simulink model "pwminverter_c"  (R2019b)
settings: Solver=ode23tb  StartTime=0.0  StopTime=0.2  RelTol=1e-3  EnableMultiTasking=on
libraries: powerlib x50, powerlib_meascontrol x1
settings Model: Creator=g0305973  LastModifiedBy=User
settings DataIOCC: LimitDataPoints=on  SaveFormat=Array  SignalLoggingSaveFormat=ModelDataLogs  ReturnWorkspaceOutputs=off
settings OptimizationCC: ExpressionDepthLimit=2147483647  InitFltsAndDblsToZero=on  LifeSpan=inf
settings DebuggingCC: SaveWithParameterizedLinksMsg=none  UnderspecifiedInitializationDetection=Classic  MergeDetectMultiDrivingBlocksExec=none  SignalResolutionControl=TryResolveAllWithWarning  SolverPrmCheckMsg=warning  FcnCallInpInsideContextMsg=warning  StateNameClashWarn=warning  SFUnexpectedBacktrackingDiag=warning  SFNoUnconditionalDefaultTransitionDiag=warning  SFExecutionAtInitializationDiag=none  ArithmeticOperatorsInVariantConditions=warning
settings HardwareCC: ProdBitPerPointer=32  ProdBitPerSizeT=32  ProdBitPerPtrDiffT=32  ProdLargestAtomicFloat=None  ProdIntDivRoundTo=Undefined  ProdEndianess=Unspecified  ProdWordSize=32  ProdHWDeviceType=32-bit Generic
settings ModelReferenceCC: PropagateSignalLabelsOutOfModel=off
settings SFSimCC: SimUseLocalCustomCode=off  CustomCodeUndefinedFunction=UseInterfaceOnly
settings RTWCC: RTWUseLocalCustomCode=off
settings CodeAppCC: StateflowObjectComments=on
settings GRTTargetCC: TargetFcnLib=ansi_tfl_tmw.mat  TargetLangStandard=C89/C90 (ANSI)  CombineOutputUpdateFcns=off  GRTInterface=on
settings ConfigComp: CovMetricSettings=dw  CovSaveCumulativeToWorkspaceVar=on  CovSaveSingleToWorkspaceVar=on  CovExternalEMLEnable=off
settings SimscapeCC: SimscapeNormalizeSystem=off

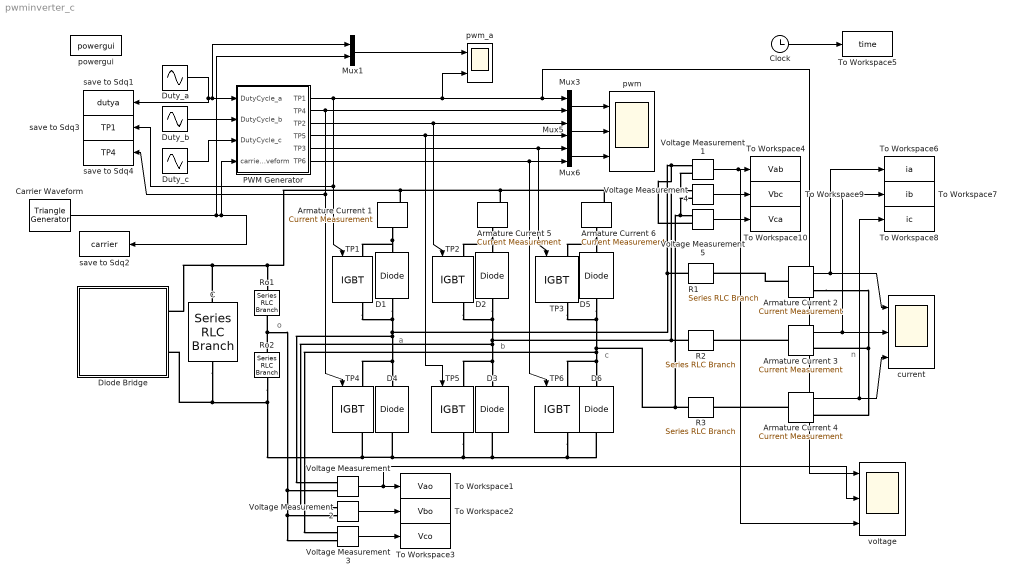
== system pwminverter_c ==
  note: o
  note: n
  note: a
  note: b
  note: c
  Armature Current {1..6} (6 alike) : powerlib/Measurements/Current Measurement  Tag=PoWeRsYsTeMmEaSuReMeNt  PhasorSimulation=off  OutputType=Magnitude  PSBequivalent=0
  C : powerlib/Elements/Series RLC Branch  LConnTagsString=__new0  RConnTagsString=__new0  BranchType=C  Resistance=1.0  Inductance=0.005  SetiL0=off  InitialCurrent=0  Capacitance=100000e-6  Setx0=on  InitialVoltage=390  Measurements=None
  Carrier Waveform : powerlib_meascontrol/Pulse & Signal Generators/Triangle Generator  Freq=2000  Phase=90  Ts=0
  Clock : Clock
  D{1..6} (6 alike) : powerlib/Power Electronics/Diode  Ron=1e-3  Lon=0  Vf=0  IC=0  UseSnubber=off  Rs=1e5  Cs=inf  Measurements=off
  Diode Bridge : Subsystem
  Duty_a : Sin  Amplitude=0.5  Frequency=200*pi  SampleTime=0
  Duty_b : Sin  Amplitude=0.5  Frequency=200*pi  Phase=-2*pi/3  SampleTime=0
  Duty_c : Sin  Amplitude=0.5  Frequency=200*pi  Phase=2*pi/3  SampleTime=0
  Mux{1,3,5..6} (4 alike) : Mux  Inputs=2
  PWM Generator : Subsystem
      mask Display: plot([1,2,2,3,3,4,4,5,5,6],[0,0,5,5,0,0,5,5,0,0])
  R1 : powerlib/Elements/Series RLC Branch  LConnTagsString=__new0  RConnTagsString=__new0  BranchType=RL  Resistance=660  Inductance=1.6  SetiL0=off  InitialCurrent=0  Capacitance=10000e-6  Setx0=off  InitialVoltage=0  Measurements=None
  R2 : powerlib/Elements/Series RLC Branch  LConnTagsString=__new0  RConnTagsString=__new0  BranchType=RL  Resistance=660  Inductance=1.6  SetiL0=off  InitialCurrent=0  Capacitance=10000e-6  Setx0=off  InitialVoltage=0  Measurements=None
  R3 : powerlib/Elements/Series RLC Branch  LConnTagsString=__new0  RConnTagsString=__new0  BranchType=RL  Resistance=660  Inductance=1.6  SetiL0=off  InitialCurrent=0  Capacitance=10000e-6  Setx0=off  InitialVoltage=0  Measurements=None
  Ro1 : powerlib/Elements/Series RLC Branch  LConnTagsString=__new0  RConnTagsString=__new0  BranchType=R  Resistance=4800  Inductance=0.005  SetiL0=off  InitialCurrent=0  Capacitance=10000e-6  Setx0=off  InitialVoltage=0  Measurements=None
  Ro2 : powerlib/Elements/Series RLC Branch  LConnTagsString=__new0  RConnTagsString=__new0  BranchType=R  Resistance=4800  Inductance=0.005  SetiL0=off  InitialCurrent=0  Capacitance=10000e-6  Setx0=off  InitialVoltage=0  Measurements=None
  TP{1..6} (6 alike) : powerlib/Power Electronics/IGBT  Ron=0.001  Lon=0  Vf=0  Tf=1e-6  Tt=2e-6  IC=0  Rs=1e5  Cs=inf  Measurements=on
  To Workspace1 : ToWorkspace  VariableName=Vao  SampleTime=1e-5
  To Workspace10 : ToWorkspace  VariableName=Vca  SampleTime=1e-5
  To Workspace2 : ToWorkspace  VariableName=Vbo  SampleTime=1e-5
  To Workspace3 : ToWorkspace  VariableName=Vco  SampleTime=1e-5
  To Workspace4 : ToWorkspace  VariableName=Vab  SampleTime=1e-5
  To Workspace5 : ToWorkspace  VariableName=time  SampleTime=1e-5
  To Workspace6 : ToWorkspace  VariableName=ia  SampleTime=1e-5
  To Workspace7 : ToWorkspace  VariableName=ib  SampleTime=1e-5
  To Workspace8 : ToWorkspace  VariableName=ic  SampleTime=1e-5
  To Workspace9 : ToWorkspace  VariableName=Vbc  SampleTime=1e-5
  Voltage Measurement{,1..5} (6 alike) : powerlib/Measurements/Voltage Measurement  PhasorSimulation=off  OutputType=Complex  PSBequivalent=0
  current : Scope  NumInputPorts=3
  powergui : powerlib/powergui  SimulationMode=Continuous  SampleTime=50e-6  frequency=60  Iterations=50  frequencyindice=50  Pbase=100e6  ErrMax=1e-4  UnitsV=kV  UnitsW=MW  buscounter=0  FunctionMessages=off  echomessages=off  EnableUseOfTLC=off  CurrentSourceSwitches=on  DisableSnubberDevices=off  DisableRonSwitches=off  DisableVfSwitches=off  DisplayEquations=off  AutomaticDiscreteSolvers=off  SolverType=Tustin  Interpol=off  ExternalGateDelay=off  methode=off  Ts=0  x0status=blocks  SPID=off  SwTol=0  HookPort=off  NonlinearTolerance=1e-4  nMaxIteration=100  ContinueOnMaxIteration=off  RestoreLinks=warning  ResistiveCurrentMeasurement=off  Frange=[0:2:500]  Ylog=off  Xlog=on  ShowGrid=off  save=off  variable=ZData  structure=PhaseCurrent  ZoomFFT=on  StartTime=0.0  cycles=10  DisplayStyle=1  fundamental=100  FreqAxis=off  MaxFrequency=3000  frequencyindicesteady=1  RmsSteady=1  display=off
  pwm : Scope  NumInputPorts=3
  pwm_a : Scope  NumInputPorts=2
  save to Sdq1 : ToWorkspace  VariableName=dutya  SampleTime=1e-5
  save to Sdq2 : ToWorkspace  VariableName=carrier  SampleTime=1e-5
  save to Sdq3 : ToWorkspace  VariableName=TP1  SampleTime=1e-5
  save to Sdq4 : ToWorkspace  VariableName=TP4  SampleTime=1e-5
  voltage : Scope  NumInputPorts=3
  wires:
  Clock/1 -> To Workspace5/1
  PWM Generator/1(TP1) -> Mux3/1, voltage/1, pwm_a/2, TP1/1, save to Sdq3/1
  PWM Generator/2(TP4) -> Mux3/2, TP4/1, save to Sdq4/1
  PWM Generator/3(TP2) -> Mux5/1, TP2/1
  PWM Generator/4(TP5) -> Mux5/2, TP5/1
  PWM Generator/5(TP3) -> Mux6/1, TP3/1
  PWM Generator/6(TP6) -> Mux6/2, TP6/1
  Duty_b/1 -> PWM Generator/2(DutyCycle_b)
  Duty_a/1 -> PWM Generator/1(DutyCycle_a), Mux1/1, save to Sdq1/1
  Duty_c/1 -> PWM Generator/3(DutyCycle_c)
  Mux3/1 -> pwm/1
  Mux5/1 -> pwm/2
  Mux6/1 -> pwm/3
  Voltage Measurement1/1 -> voltage/3, To Workspace4/1
  Voltage Measurement/1 -> voltage/2, To Workspace1/1
  Carrier Waveform/1 -> save to Sdq2/1, PWM Generator/4(carrier waveform), Mux1/2
  Mux1/1 -> pwm_a/1
  Voltage Measurement2/1 -> To Workspace2/1
  Voltage Measurement3/1 -> To Workspace3/1
  Armature Current 3/1 -> current/2, To Workspace7/1
  Armature Current 4/1 -> current/3, To Workspace8/1
  Voltage Measurement4/1 -> To Workspace9/1
  Voltage Measurement5/1 -> To Workspace10/1
  Armature Current 2/1 -> current/1, To Workspace6/1
  connections:
  Armature Current 2/LConn1 -- R1/LConn1
  Armature Current 3/LConn1 -- R2/LConn1
  Armature Current 4/LConn1 -- R3/LConn1
  Armature Current 2/RConn1 -- Armature Current 3/RConn1 -- Armature Current 4/RConn1
  Ro2/LConn1 -- Ro1/RConn1 -- Voltage Measurement/LConn2 -- Voltage Measurement2/LConn2 -- Voltage Measurement3/LConn2
  R3/RConn1 -- TP3/RConn1 -- D5/LConn1 -- TP6/LConn1 -- D6/RConn1 -- Voltage Measurement3/LConn1 -- Voltage Measurement4/LConn2 -- Voltage Measurement5/LConn1
  R2/RConn1 -- TP2/RConn1 -- D2/LConn1 -- D3/RConn1 -- TP5/LConn1 -- Voltage Measurement2/LConn1 -- Voltage Measurement1/LConn2 -- Voltage Measurement4/LConn1
  R1/RConn1 -- TP4/LConn1 -- D4/RConn1 -- Voltage Measurement/LConn1 -- TP1/RConn1 -- D1/LConn1 -- Voltage Measurement5/LConn2 -- Voltage Measurement1/LConn1
  D5/RConn1 -- Armature Current 6/LConn1 -- TP3/LConn1
  D2/RConn1 -- Armature Current 5/LConn1 -- TP2/LConn1
  Armature Current 6/RConn1 -- C/LConn1 -- Diode Bridge/LConn1 -- Ro1/LConn1 -- Armature Current 1/RConn1 -- Armature Current 5/RConn1
  TP1/LConn1 -- Armature Current 1/LConn1 -- D1/RConn1
  C/RConn1 -- Diode Bridge/LConn2 -- D4/LConn1 -- TP5/RConn1 -- TP6/RConn1 -- D6/LConn1 -- D3/LConn1 -- TP4/RConn1 -- Ro2/RConn1

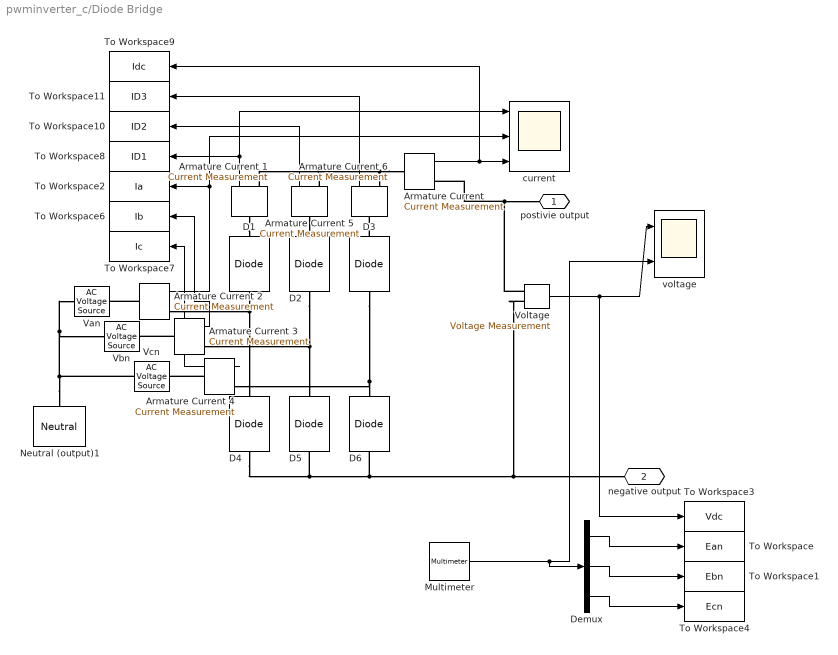
== system pwminverter_c/Diode Bridge ==
  Armature Current {,1..6} (7 alike) : powerlib/Measurements/Current Measurement  Tag=PoWeRsYsTeMmEaSuReMeNt  PhasorSimulation=off  OutputType=Magnitude  PSBequivalent=0
  D{1..6} (6 alike) : powerlib/Power Electronics/Diode  Ron=1e-3  Lon=0  Vf=0  IC=0  UseSnubber=off  Rs=1e5  Cs=inf  Measurements=off
  Demux : Demux  Outputs=3
      settings: DisplayOption=none
  Multimeter : powerlib/Measurements/Multimeter  PhasorSimulation=off  OutputType=Complex  sel=[1 2 3]  L=3  Gain=[1 1 1]  yselected={'Usrc: Diode Bridge/Van','Usrc: Diode Bridge/Vbn','Usrc: Diode Bridge/Vcn'};  PSBOutputType=1  PSBequivalent=0  AxesSetting=[0,0.1,-100,100]  Display=0  SavedBlockNames=-11
  Neutral (output)1 : powerlib/Elements/Neutral  LConnTagsString=a  NodeNumber=99
      settings: SourceProductBaseCode=PS
  To Workspace : ToWorkspace  VariableName=Ean  SampleTime=1e-4
  To Workspace1 : ToWorkspace  VariableName=Ebn  SampleTime=1e-4
  To Workspace10 : ToWorkspace  VariableName=ID2  SampleTime=1e-4
  To Workspace11 : ToWorkspace  VariableName=ID3  SampleTime=1e-4
  To Workspace2 : ToWorkspace  VariableName=Ia  SampleTime=1e-4
  To Workspace3 : ToWorkspace  VariableName=Vdc  SampleTime=1e-4
  To Workspace4 : ToWorkspace  VariableName=Ecn  SampleTime=1e-4
  To Workspace6 : ToWorkspace  VariableName=Ib  SampleTime=1e-4
  To Workspace7 : ToWorkspace  VariableName=Ic  SampleTime=1e-4
  To Workspace8 : ToWorkspace  VariableName=ID1  SampleTime=1e-4
  To Workspace9 : ToWorkspace  VariableName=Idc  SampleTime=1e-4
  Van : powerlib/Electrical Sources/AC Voltage Source  Description=source block  Amplitude=240*1.414  Phase=0  Frequency=50  SampleTime=0  Measurements=Voltage  BusType=swing  Pref=10e3  Qref=0  Qmin=-inf  Qmax=+inf
      settings: AttributesFormatString=\n
  Vbn : powerlib/Electrical Sources/AC Voltage Source  Description=source block  Amplitude=240*1.414  Phase=-120  Frequency=50  SampleTime=0  Measurements=Voltage  BusType=swing  Pref=10e3  Qref=0  Qmin=-inf  Qmax=+inf
      settings: AttributesFormatString=\n
  Vcn : powerlib/Electrical Sources/AC Voltage Source  Description=source block  Amplitude=240*1.414  Phase=120  Frequency=50  SampleTime=0  Measurements=Voltage  BusType=swing  Pref=10e3  Qref=0  Qmin=-inf  Qmax=+inf
      settings: AttributesFormatString=\n
  "Voltage " : powerlib/Measurements/Voltage Measurement  PhasorSimulation=off  OutputType=Complex  PSBequivalent=0
  current : Scope  NumInputPorts=3
  voltage : Scope  NumInputPorts=2
  postivie output : PMIOPort  Side=Left
  negative output : PMIOPort  Port=2  Side=Left
  wires:
  Armature Current 6/1 -> To Workspace11/1
  Armature Current 5/1 -> To Workspace10/1
  Armature Current 4/1 -> To Workspace7/1
  Armature Current 3/1 -> To Workspace6/1
  "Armature Current "/1 -> To Workspace9/1, current/3
  Armature Current 2/1 -> To Workspace2/1, current/2
  Armature Current 1/1 -> To Workspace8/1, current/1
  Demux/1 -> To Workspace/1
  Demux/2 -> To Workspace1/1
  Demux/3 -> To Workspace4/1
  Multimeter/1 -> voltage/2, Demux/1
  "Voltage "/1 -> voltage/1, To Workspace3/1
  connections:
  "Armature Current "/LConn1 -- Armature Current 1/RConn1 -- Armature Current 5/RConn1 -- Armature Current 6/RConn1
  "Armature Current "/RConn1 -- "Voltage "/LConn1 -- postivie output/RConn1
  Armature Current 1/LConn1 -- D1/RConn1
  Armature Current 2/LConn1 -- Van/RConn1
  Armature Current 2/RConn1 -- D4/RConn1 -- D1/LConn1
  Armature Current 3/LConn1 -- Vbn/RConn1
  Armature Current 3/RConn1 -- D5/RConn1 -- D2/LConn1
  Armature Current 4/LConn1 -- Vcn/RConn1
  Armature Current 4/RConn1 -- D3/LConn1 -- D6/RConn1
  Armature Current 5/LConn1 -- D2/RConn1
  D3/RConn1 -- Armature Current 6/LConn1
  D6/LConn1 -- D5/LConn1 -- D4/LConn1 -- negative output/RConn1 -- "Voltage "/LConn2
  Neutral (output)1/LConn1 -- Vbn/LConn1 -- Van/LConn1 -- Vcn/LConn1

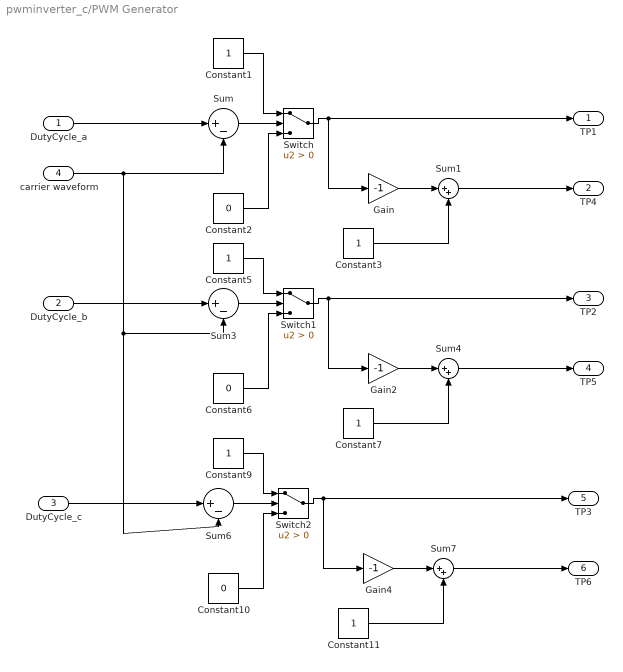
== system pwminverter_c/PWM Generator ==
  DutyCycle_a : Inport
  DutyCycle_b : Inport  Port=2
  DutyCycle_c : Inport  Port=3
  carrier waveform : Inport  Port=4
  Constant{1,3,5,7,9,11} (6 alike) : Constant
  Constant10 : Constant  Value=0
  Constant2 : Constant  Value=0
  Constant6 : Constant  Value=0
  Gain : Gain  Gain=-1  SaturateOnIntegerOverflow=on  OutDataTypeStr=Inherit: Same as input  ParamDataTypeStr=Inherit: Same as input
  Gain2 : Gain  Gain=-1  SaturateOnIntegerOverflow=on  OutDataTypeStr=Inherit: Same as input  ParamDataTypeStr=Inherit: Same as input
  Gain4 : Gain  Gain=-1  SaturateOnIntegerOverflow=on  OutDataTypeStr=Inherit: Same as input  ParamDataTypeStr=Inherit: Same as input
  Sum : Sum  Inputs=|+-  SaturateOnIntegerOverflow=on
  Sum1 : Sum  Inputs=|++  SaturateOnIntegerOverflow=on
  Sum3 : Sum  Inputs=|+-  SaturateOnIntegerOverflow=on
  Sum4 : Sum  Inputs=|++  SaturateOnIntegerOverflow=on
  Sum6 : Sum  Inputs=|+-  SaturateOnIntegerOverflow=on
  Sum7 : Sum  Inputs=|++  SaturateOnIntegerOverflow=on
  Switch : Switch  Criteria=u2 > Threshold  SaturateOnIntegerOverflow=on
  Switch1 : Switch  Criteria=u2 > Threshold  SaturateOnIntegerOverflow=on
  Switch2 : Switch  Criteria=u2 > Threshold  SaturateOnIntegerOverflow=on
  TP1 : Outport
  TP4 : Outport  Port=2
  TP2 : Outport  Port=3
  TP5 : Outport  Port=4
  TP3 : Outport  Port=5
  TP6 : Outport  Port=6
  wires:
  Constant3/1 -> Sum1/2
  Gain/1 -> Sum1/1
  Switch/1 -> TP1/1, Gain/1
  Constant2/1 -> Switch/3
  Constant1/1 -> Switch/1
  Sum/1 -> Switch/2
  Sum1/1 -> TP4/1
  carrier waveform/1 -> Sum/2, Sum3/2, Sum6/2
  DutyCycle_a/1 -> Sum/1
  Constant7/1 -> Sum4/2
  Gain2/1 -> Sum4/1
  Switch1/1 -> Gain2/1, TP2/1
  Constant6/1 -> Switch1/3
  Constant5/1 -> Switch1/1
  Sum3/1 -> Switch1/2
  Sum4/1 -> TP5/1
  DutyCycle_b/1 -> Sum3/1
  Constant11/1 -> Sum7/2
  Gain4/1 -> Sum7/1
  Switch2/1 -> TP3/1, Gain4/1
  Constant10/1 -> Switch2/3
  Constant9/1 -> Switch2/1
  Sum6/1 -> Switch2/2
  Sum7/1 -> TP6/1
  DutyCycle_c/1 -> Sum6/1
